simulink model "HighpassFilter"  (R2020a)
settings: Solver=VariableStepAuto  StartTime=0.0  StopTime=10.0  RelTol=1e-3
settings Model: Creator=Shubham  LastModifiedBy=Shubham
settings DataIOCC: SaveOutput=off  SaveTime=off

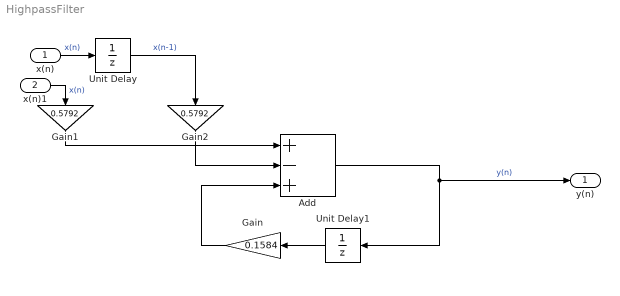
== system HighpassFilter ==
  x(n) : Inport  OutDataTypeStr=double  PortDimensions=1  SampleTime=0
  x(n)1 : Inport  Port=2  OutDataTypeStr=double  PortDimensions=1  SampleTime=0
  Add : Sum  Inputs=+-+
  Gain : Gain  Gain=0.1584
  Gain1 : Gain  Gain=0.5792
  Gain2 : Gain  Gain=0.5792
  Unit Delay : UnitDelay  InitialCondition=1  SampleTime=-1  HasFrameUpgradeWarning=on
  Unit Delay1 : UnitDelay  SampleTime=-1  HasFrameUpgradeWarning=on
  y(n) : Outport  OutDataTypeStr=double  PortDimensions=1  SampleTime=0
  wires:
  Unit Delay1/1 -> Gain/1
  Unit Delay/1 -> Gain2/1  "x(n-1)"
  Add/1 -> Unit Delay1/1, y(n)/1  "y(n)"
  x(n)/1 -> Unit Delay/1  "x(n)"
  x(n)1/1 -> Gain1/1  "x(n)"
  Gain/1 -> Add/3
  Gain1/1 -> Add/1
  Gain2/1 -> Add/2
